simulink model "j53"  (R2015b)
settings: Solver=VariableStepAuto  StartTime=-10  StopTime=10  RelTol=1e-3
libraries: simulink x1
settings Model: Creator=Pouya  LastModifiedBy=Pouya

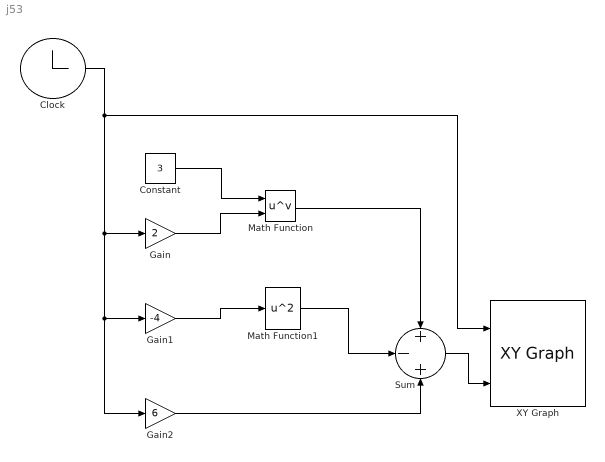
== system j53 ==
  Clock : Clock
  Constant : Constant  Value=3
  Gain : Gain  Gain=2
  Gain1 : Gain  Gain=-4
  Gain2 : Gain  Gain=6
  Math Function : Math  Operator=pow  SaturateOnIntegerOverflow=on
  Math Function1 : Math  Operator=square  SaturateOnIntegerOverflow=on
  Sum : Sum  Inputs=+-+
  XY Graph : simulink/Sinks/XY Graph  xmin=-10  xmax=10  ymin=-100  ymax=100  st=-1
  wires:
  Gain/1 -> Math Function/2
  Constant/1 -> Math Function/1
  Sum/1 -> XY Graph/2
  Math Function/1 -> Sum/1
  Gain1/1 -> Math Function1/1
  Gain2/1 -> Sum/3
  Math Function1/1 -> Sum/2
  Clock/1 -> Gain2/1, Gain1/1, Gain/1, XY Graph/1
